simulink model "simulink_1"  (R2018b)
settings: Solver=VariableStepAuto  StartTime=0.0  StopTime=10.0  RelTol=1e-3
values from neighbouring files (symbols this model uses):
  B = 12    [mass_spring.m]
  k = 16    [mass_spring.m]
  m = 2    [mass_spring.m]
  x0 = 3    [mass_spring.m]
settings Model: Creator=student  LastModifiedBy=pal35

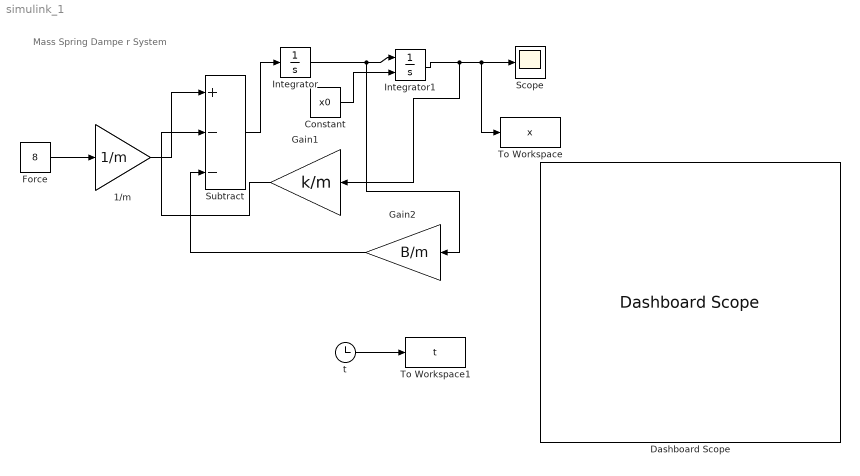
== system simulink_1 ==
  note: Mass Spring Dampe r System
  1/m : Gain  Gain=1/m
  Constant : Constant  Value=x0
  Dashboard Scope : DashboardScope  WebBlockId=14  Ymin=5  Ymax=8
  Force : Constant  Value=8
  Gain1 : Gain  Gain=k/m
  Gain2 : Gain  Gain=B/m
  Integrator : Integrator
  Integrator1 : Integrator  InitialConditionSource=external  InitialCondition=5
  Scope : Scope
  Subtract : Sum  Inputs=+--
  To Workspace : ToWorkspace  VariableName=x  SaveFormat=Timeseries  SampleTime=-1
  To Workspace1 : ToWorkspace  VariableName=t  SaveFormat=Timeseries  SampleTime=-1
  t : Clock
  wires:
  Integrator/1 -> Gain2/1, Integrator1/1
  Force/1 -> 1/m/1
  1/m/1 -> Subtract/1
  Gain1/1 -> Subtract/2
  Gain2/1 -> Subtract/3
  Subtract/1 -> Integrator/1
  Integrator1/1 -> To Workspace/1, Scope/1, Gain1/1
  Constant/1 -> Integrator1/2
  t/1 -> To Workspace1/1
